simulink library "ddm"  (R2021b)
settings: Solver=VariableStepAuto  StartTime=0.0  StopTime=10.0  RelTol=1e-3
undefined symbols (not defined in the file or in its folder): ENUM_ADASACCSTA_ERROR, ENUM_ADASACCSTA_OFF, ENUM_ADASACCSTA_STANDBY, ENUM_ADASISASTA_OFF, ENUM_ALLOWMOV_ALLOWREADY, ENUM_APS, ENUM_BRKSTA_ERROR, ENUM_BRKSTA_OFF, ENUM_BRKSTA_ON, ENUM_CHGPREACTERRSTA_OBCPRE, ENUM_DCDCFAULTSTA_ANYFAULTLV1, ENUM_DCDCFAULTSTA_ANYFAULTLV2, ENUM_DRIVETRAIN_AWD, ENUM_DRIVETRAIN_FWD, ENUM_DRIVETRAIN_RWD, ENUM_DRSEATSTA_INVALID, ENUM_EDUDRTSTA_NORMAL, ENUM_EPBSTA_APPLIED, ENUM_EPBSTA_RELEASED, ENUM_HVBATTREADYPRE_READY, ENUM_MCUWARN_LV0, ENUM_MCUWARN_LV1, ENUM_MCUWARN_LV2, ENUM_MCUWARN_LV3, ENUM_MCUWARN_NOERROR, ENUM_OBCFAULTSTA_ANYFAULT, ENUM_PAS_R2F2, ENUM_PDFAULT_BATTPDFAIL, ENUM_PDFAULT_DCDCDISABLE, ENUM_PDFAULT_MCUDISABLE, ENUM_PDFAULT_MCUDISCHRG, ENUM_POWERSTA_OFF, ENUM_POWERSTA_ON, ENUM_POWERSTA_READY, ENUM_POWERSTA_STANDBY, ENUM_PRESSINDI_LOW, ENUM_PUFAULT_BATTUPFAIL, ENUM_PUFAULT_DCDCENABLEFAIL, ENUM_PUFAULT_PRECHRGCHKFAIL, ENUM_PUFAULT_SAFETYCHKFAIL, ENUM_PUSTATE_COMPLETED, ENUM_PWRSTASW_OFF, ENUM_PWRSTASW_OFFA, ENUM_PWRSTASW_OFFCHVCHRG, ENUM_PWRSTASW_OFFCLVCHRG, ENUM_PWRSTASW_ON, ENUM_PWRSTASW_ONHVCHRG, ENUM_PWRSTASW_READY, ENUM_PWRSTASW_STANDBY, ENUM_RANGESTA_12IN, ENUM_RANGESTA_12OUT, ENUM_SHIFTCOMMAND_D, ENUM_SHIFTCOMMAND_N, ENUM_SHIFTCOMMAND_P, ENUM_SHIFTCOMMAND_R, ENUM_ZONEMALFUNLV_1ST, ENUM_ZONEMALFUNLV_2ND, ENUM_ZONEMALFUNLV_3RD, ENUM_ZONEMALFUNLV_4TH, ENUM_ZONESPDCTRLMODE_ACC ... (+832)
libraries: hcu_lib x738, $bdroot x26, simulink x7
(part 4 of 25)

== system ddm/DDM/DDM/TQD ==
  VPMM_SysPwrSta_enum : Inport
  VINP_AccelPedal1Vol_V : Inport  Port=2
  VINP_AccelPedal2Vol_V : Inport  Port=3
  VDHP_EAPS12RangeSta_enum : Inport  Port=4
  VDHP_EAPCRBAD_flg : Inport  Port=5
  task_time_s : Inport  Port=6
  DTC_clear_request : Inport  Port=7
  No_CAN3_BUS_OFF : Inport  Port=8
  No_CAN1_BUS_OFF : Inport  Port=9
  VINP_CANMsgValidMCUF1_flg : Inport  Port=10
  VINP_CANMsgValidMCUR1_flg : Inport  Port=11
  VINP_CANMsgValidShifter1_flg : Inport  Port=12
  VINP_CANMsgValidESC7_flg : Inport  Port=13
  VINP_CANMsgValidESC1_flg : Inport  Port=14
  VINP_CANMsgValidESC5_flg : Inport  Port=15
  VDDM_MCUF1RCErr_flg : Inport  Port=16
  VDDM_MCUF1CSErr_flg : Inport  Port=17
  VDDM_MCUR1RCErr_flg : Inport  Port=18
  VDDM_MCUR1CSErr_flg : Inport  Port=19
  VDDM_Shifter1RCErr_flg : Inport  Port=20
  VDDM_Shifter1CSErr_flg : Inport  Port=21
  VDDM_ESC7RCErr_flg : Inport  Port=22
  VDDM_ESC7CSErr_flg : Inport  Port=23
  VDDM_ESC1RCErr_flg : Inport  Port=24
  VDDM_ESC1CSErr_flg : Inport  Port=25
  VDDM_ESC5RCErr_flg : Inport  Port=26
  VDDM_ESC5CSErr_flg : Inport  Port=27
  VINP_FrEDUDrtSta_flg : Inport  Port=28
  VINP_VehSpeed_kph : Inport  Port=29
  VINP_FrEDURealTMTq_Nm : Inport  Port=30
  VTQR_FrTMTqReq_Nm : Inport  Port=31
  VINP_RrEDUDrtSta_flg : Inport  Port=32
  VINP_RrEDURealTMTq_Nm : Inport  Port=33
  VTQR_RrTMTqReq_Nm : Inport  Port=34
  VINP_MCUWarnF_enum : Inport  Port=35
  VINP_MCUWarnR_enum : Inport  Port=36
  APS_DDM : Subsystem
  EPB : Subsystem  Commented=on
  ESC1_DDM : Subsystem
  ESC5_DDM : Subsystem
  ESC7_DDM : Subsystem
  Logical Operator{,1..5} (6 alike) : Logic  Operator=NOT  AllPortsSameDT=off  OutDataTypeStr=boolean
  MCU1_DDM : Subsystem
  MCU_DDM : Subsystem
  Shifter1_DDM : Subsystem
  VDDM_APS1SigOoRDTC_raw32 : Outport
  VDDM_APS2SigOoRDTC_raw32 : Outport  Port=2
  VDDM_APSCorrErrDTC_raw32 : Outport  Port=3
  VDDM_MCUF1NoComDTC_raw32 : Outport  Port=4
  VDDM_MCUR1NoComDTC_raw32 : Outport  Port=5
  VDDM_Shifter1NoComDTC_raw32 : Outport  Port=6
  VDDM_ESC7NoComDTC_raw32 : Outport  Port=7
  VDDM_ESC1NoComDTC_raw32 : Outport  Port=8
  VDDM_ESC5NoComDTC_raw32 : Outport  Port=9
  VDDM_MCUF1RCErrDTC_raw32 : Outport  Port=10
  VDDM_MCUR1RCErrDTC_raw32 : Outport  Port=11
  VDDM_MCUF1CSErrDTC_raw32 : Outport  Port=12
  VDDM_MCUR1CSErrDTC_raw32 : Outport  Port=13
  VDDM_Shifter1RCErrDTC_raw32 : Outport  Port=14
  VDDM_Shifter1CSErrDTC_raw32 : Outport  Port=15
  VDDM_ESC7RCErrDTC_raw32 : Outport  Port=16
  VDDM_ESC7CSErrDTC_raw32 : Outport  Port=17
  VDDM_ESC1RCErrDTC_raw32 : Outport  Port=18
  VDDM_ESC1CSErrDTC_raw32 : Outport  Port=19
  VDDM_ESC5RCErrDTC_raw32 : Outport  Port=20
  VDDM_ESC5CSErrDTC_raw32 : Outport  Port=21
  VDDM_FrMCUTqErrDTC_raw32 : Outport  Port=22
  VDDM_RrMCUTqErrDTC_raw32 : Outport  Port=23
  VDDM_MCUF1NoComCFS_flg : Outport  Port=24
  VDDM_MCUF1RCErrCFS_flg : Outport  Port=25
  VDDM_MCUF1CSErrCFS_flg : Outport  Port=26
  VDDM_MCUR1NoComCFS_flg : Outport  Port=27
  VDDM_MCUR1RCErrCFS_flg : Outport  Port=28
  VDDM_MCUR1CSErrCFS_flg : Outport  Port=29
  VDDM_ESC7NoComCFS_flg : Outport  Port=30
  VDDM_ESC7RCErrCFS_flg : Outport  Port=31
  VDDM_ESC7CSErrCFS_flg : Outport  Port=32
  VDDM_ESC1NoComCFS_flg : Outport  Port=33
  VDDM_ESC1RCErrCFS_flg : Outport  Port=34
  VDDM_ESC1CSErrCFS_flg : Outport  Port=35
  VDDM_ESC5NoComCFS_flg : Outport  Port=36
  VDDM_ESC5RCErrCFS_flg : Outport  Port=37
  VDDM_ESC5CSErrCFS_flg : Outport  Port=38
  wires:
  VINP_AccelPedal2Vol_V/1 -> [VINP_AccelPedal2Vol_V]
  VDHP_EAPS12RangeSta_enum/1 -> [VDHP_EAPS12RangeSta_enum]
  VDHP_EAPCRBAD_flg/1 -> [VDHP_EAPCRBAD_flg]
  VINP_AccelPedal1Vol_V/1 -> [VINP_AccelPedal1Vol_V]
  VPMM_SysPwrSta_enum/1 -> [VPMM_SysPwrSta_enum]
  [VDHP_EAPCRBAD_flg] -> APS_DDM/5(VDHP_EAPCRBAD_flg)
  [VPMM_SysPwrSta_enum] -> APS_DDM/1(VPMM_SysPwrSta_enum)
  [VINP_AccelPedal1Vol_V] -> APS_DDM/2(VINP_AccelPedal1Vol_V)
  [VINP_AccelPedal2Vol_V] -> APS_DDM/3(VINP_AccelPedal2Vol_V)
  [VDHP_EAPS12RangeSta_enum] -> APS_DDM/4(VDHP_EAPS12RangeSta_enum)
  APS_DDM/1(VDDM_APS1SigOoRDTC_raw32) -> VDDM_APS1SigOoRDTC_raw32/1
  APS_DDM/2(VDDM_APS2SigOoRDTC_raw32) -> VDDM_APS2SigOoRDTC_raw32/1
  APS_DDM/3(VDDM_APSCorrErrDTC_raw32) -> VDDM_APSCorrErrDTC_raw32/1
  task_time_s/1 -> [task_time_s]
  [task_time_s] -> APS_DDM/6(task_time_s)
  DTC_clear_request/1 -> [DTC_clear_request]
  [DTC_clear_request] -> APS_DDM/7(DTC_clear_request)
  [task_time_s] -> MCU1_DDM/1(task_time_s)
  [task_time_s] -> Shifter1_DDM/1(task_time_s)
  [task_time_s] -> ESC7_DDM/1(task_time_s)
  [VPMM_SysPwrSta_enum] -> MCU1_DDM/2(VPMM_SysPwrSta_enum)
  [No_CAN3_BUS_OFF] -> MCU1_DDM/3(No_CAN3_BUS_OFF)
  [VDDM_MCUF1NoCom_flg] -> MCU1_DDM/4(VDDM_MCUF1NoCom_flg)
  [VDDM_MCUR1NoCom_flg] -> MCU1_DDM/5(VDDM_MCUR1NoCom_flg)
  [DTC_clear_request] -> MCU1_DDM/10(DTC_clear_request)
  [VPMM_SysPwrSta_enum] -> Shifter1_DDM/2(VPMM_SysPwrSta_enum)
  [No_CAN3_BUS_OFF] -> Shifter1_DDM/3(No_CAN3_BUS_OFF)
  [VDDM_Shifter1NoCom_flg] -> Shifter1_DDM/4(VDDM_Shifter1NoCom_flg)
  [DTC_clear_request] -> Shifter1_DDM/7(DTC_clear_request)
  [VDDM_ESC7NoCom_flg] -> ESC7_DDM/4(VDDM_ESC7NoCom_flg)
  [No_CAN1_BUS_OFF] -> ESC7_DDM/3(No_CAN1_BUS_OFF)
  [VPMM_SysPwrSta_enum] -> ESC7_DDM/2(VPMM_SysPwrSta_enum)
  [DTC_clear_request] -> ESC7_DDM/7(DTC_clear_request)
  [task_time_s] -> ESC1_DDM/1(task_time_s)
  [VPMM_SysPwrSta_enum] -> ESC1_DDM/2(VPMM_SysPwrSta_enum)
  [No_CAN1_BUS_OFF] -> ESC1_DDM/3(No_CAN1_BUS_OFF)
  [VDDM_ESC1NoCom_flg] -> ESC1_DDM/4(VDDM_ESC1NoCom_flg)
  [DTC_clear_request] -> ESC1_DDM/7(DTC_clear_request)
  [task_time_s] -> ESC5_DDM/1(task_time_s)
  [VPMM_SysPwrSta_enum] -> ESC5_DDM/2(VPMM_SysPwrSta_enum)
  [No_CAN1_BUS_OFF] -> ESC5_DDM/3(No_CAN1_BUS_OFF)
  [VDDM_ESC5NoCom_flg] -> ESC5_DDM/4(VDDM_ESC5NoCom_flg)
  [DTC_clear_request] -> ESC5_DDM/7(DTC_clear_request)
  MCU1_DDM/1(VDDM_MCUF1NoComDTC_raw32) -> VDDM_MCUF1NoComDTC_raw32/1
  MCU1_DDM/2(VDDM_MCUR1NoComDTC_raw32) -> VDDM_MCUR1NoComDTC_raw32/1
  Shifter1_DDM/1(VDDM_Shifter1NoComDTC_raw32) -> VDDM_Shifter1NoComDTC_raw32/1
  ESC1_DDM/1(VDDM_ESC1NoComDTC_raw32) -> VDDM_ESC1NoComDTC_raw32/1
  ESC5_DDM/1(VDDM_ESC5NoComDTC_raw32) -> VDDM_ESC5NoComDTC_raw32/1
  No_CAN3_BUS_OFF/1 -> [No_CAN3_BUS_OFF]
  No_CAN1_BUS_OFF/1 -> [No_CAN1_BUS_OFF]
  VINP_CANMsgValidMCUF1_flg/1 -> Logical Operator5/1
  VINP_CANMsgValidMCUR1_flg/1 -> Logical Operator4/1
  VINP_CANMsgValidShifter1_flg/1 -> Logical Operator3/1
  VINP_CANMsgValidESC7_flg/1 -> Logical Operator2/1
  VINP_CANMsgValidESC1_flg/1 -> Logical Operator1/1
  VINP_CANMsgValidESC5_flg/1 -> Logical Operator/1
  Logical Operator/1 -> [VDDM_ESC5NoCom_flg]
  Logical Operator1/1 -> [VDDM_ESC1NoCom_flg]
  Logical Operator2/1 -> [VDDM_ESC7NoCom_flg]
  Logical Operator3/1 -> [VDDM_Shifter1NoCom_flg]
  Logical Operator4/1 -> [VDDM_MCUR1NoCom_flg]
  Logical Operator5/1 -> [VDDM_MCUF1NoCom_flg]
  [VDDM_MCUF1RCErr_flg] -> MCU1_DDM/6(VDDM_MCUF1RCErr_flg)
  [VDDM_MCUF1CSErr_flg] -> MCU1_DDM/7(VDDM_MCUF1CSErr_flg)
  [VDDM_MCUR1RCErr_flg] -> MCU1_DDM/8(VDDM_MCUR1RCErr_flg)
  [VDDM_MCUR1CSErr_flg] -> MCU1_DDM/9(VDDM_MCUR1CSErr_flg)
  ESC7_DDM/1(VDDM_ESC7NoComDTC_raw32) -> VDDM_ESC7NoComDTC_raw32/1
  MCU1_DDM/4(VDDM_MCUR1RCErrDTC_raw32) -> VDDM_MCUR1RCErrDTC_raw32/1
  MCU1_DDM/3(VDDM_MCUF1RCErrDTC_raw32) -> VDDM_MCUF1RCErrDTC_raw32/1
  MCU1_DDM/5(VDDM_MCUF1CSErrDTC_raw32) -> VDDM_MCUF1CSErrDTC_raw32/1
  MCU1_DDM/6(VDDM_MCUR1CSErrDTC_raw32) -> VDDM_MCUR1CSErrDTC_raw32/1
  Shifter1_DDM/2(VDDM_Shifter1RCErrDTC_raw32) -> VDDM_Shifter1RCErrDTC_raw32/1
  Shifter1_DDM/3(VDDM_Shifter1CSErrDTC_raw32) -> VDDM_Shifter1CSErrDTC_raw32/1
  ESC7_DDM/2(VDDM_ESC7RCErrDTC_raw32) -> VDDM_ESC7RCErrDTC_raw32/1
  ESC7_DDM/3(VDDM_ESC7CSErrDTC_raw32) -> VDDM_ESC7CSErrDTC_raw32/1
  ESC1_DDM/3(VDDM_ESC1CSErrDTC_raw32) -> VDDM_ESC1CSErrDTC_raw32/1
  ESC1_DDM/2(VDDM_ESC1RCErrDTC_raw32) -> VDDM_ESC1RCErrDTC_raw32/1
  ESC5_DDM/2(VDDM_ESC5RCErrDTC_raw32) -> VDDM_ESC5RCErrDTC_raw32/1
  ESC5_DDM/3(VDDM_ESC5CSErrDTC_raw32) -> VDDM_ESC5CSErrDTC_raw32/1
  MCU_DDM/2(VDDM_RrMCUTqErrDTC_raw32) -> VDDM_RrMCUTqErrDTC_raw32/1
  MCU_DDM/1(VDDM_FrMCUTqErrDTC_raw32) -> VDDM_FrMCUTqErrDTC_raw32/1
  [VDDM_Shifter1RCErr_flg] -> Shifter1_DDM/5(VDDM_Shifter1RCErr_flg)
  [VDDM_Shifter1CSErr_flg] -> Shifter1_DDM/6(VDDM_Shifter1CSErr_flg)
  VDDM_MCUR1RCErr_flg/1 -> [VDDM_MCUR1RCErr_flg]
  VDDM_MCUR1CSErr_flg/1 -> [VDDM_MCUR1CSErr_flg]
  VDDM_MCUF1CSErr_flg/1 -> [VDDM_MCUF1CSErr_flg]
  VDDM_MCUF1RCErr_flg/1 -> [VDDM_MCUF1RCErr_flg]
  VDDM_Shifter1RCErr_flg/1 -> [VDDM_Shifter1RCErr_flg]
  VDDM_Shifter1CSErr_flg/1 -> [VDDM_Shifter1CSErr_flg]
  [VDDM_ESC7RCErr_flg] -> ESC7_DDM/5(VDDM_ESC7RCErr_flg)
  [VDDM_ESC7CSErr_flg] -> ESC7_DDM/6(VDDM_ESC7CSErr_flg)
  VDDM_ESC7CSErr_flg/1 -> [VDDM_ESC7CSErr_flg]
  VDDM_ESC7RCErr_flg/1 -> [VDDM_ESC7RCErr_flg]
  [VDDM_ESC1RCErr_flg] -> ESC1_DDM/5(VDDM_ESC1RCErr_flg)
  [VDDM_ESC1CSErr_flg] -> ESC1_DDM/6(VDDM_ESC1CSErr_flg)
  VDDM_ESC1CSErr_flg/1 -> [VDDM_ESC1CSErr_flg]
  VDDM_ESC1RCErr_flg/1 -> [VDDM_ESC1RCErr_flg]
  [VDDM_ESC5RCErr_flg] -> ESC5_DDM/5(VDDM_ESC5RCErr_flg)
  [VDDM_ESC5CSErr_flg] -> ESC5_DDM/6(VDDM_ESC5CSErr_flg)
  VDDM_ESC5CSErr_flg/1 -> [VDDM_ESC5CSErr_flg]
  VDDM_ESC5RCErr_flg/1 -> [VDDM_ESC5RCErr_flg]
  VINP_RrEDURealTMTq_Nm/1 -> [VINP_RrEDURealTMTq_Nm]
  VINP_FrEDUDrtSta_flg/1 -> [VINP_FrEDUDrtSta_flg]
  VTQR_RrTMTqReq_Nm/1 -> [VTQR_RrTMTqReq_Nm]
  VINP_FrEDURealTMTq_Nm/1 -> [VINP_FrEDURealTMTq_Nm]
  VTQR_FrTMTqReq_Nm/1 -> [VTQR_FrTMTqReq_Nm]
  VINP_RrEDUDrtSta_flg/1 -> [VINP_RrEDUDrtSta_flg]
  VINP_VehSpeed_kph/1 -> [VINP_VehSpeed_kph]
  ESC7_DDM/6(VDDM_ESC7CSErrCFS_flg) -> VDDM_ESC7CSErrCFS_flg/1
  ESC7_DDM/5(VDDM_ESC7RCErrCFS_flg) -> VDDM_ESC7RCErrCFS_flg/1
  ESC7_DDM/4(VDDM_ESC7NoComCFS_flg) -> VDDM_ESC7NoComCFS_flg/1
  ESC5_DDM/6(VDDM_ESC5CSErrCFS_flg) -> VDDM_ESC5CSErrCFS_flg/1
  ESC5_DDM/4(VDDM_ESC5NoComCFS_flg) -> VDDM_ESC5NoComCFS_flg/1
  ESC1_DDM/5(VDDM_ESC1RCErrCFS_flg) -> VDDM_ESC1RCErrCFS_flg/1
  ESC5_DDM/5(VDDM_ESC5RCErrCFS_flg) -> VDDM_ESC5RCErrCFS_flg/1
  ESC1_DDM/4(VDDM_ESC1NoComCFS_flg) -> VDDM_ESC1NoComCFS_flg/1
  ESC1_DDM/6(VDDM_ESC1CSErrCFS_flg) -> VDDM_ESC1CSErrCFS_flg/1
  VINP_MCUWarnF_enum/1 -> [VINP_MCUWarnF_enum]
  VINP_MCUWarnR_enum/1 -> [VINP_MCUWarnR_enum]
  MCU1_DDM/12(VDDM_MCUR1CSErrCFS_flg) -> [VDDM_MCUR1CSErrCFS_flg]
  MCU1_DDM/8(VDDM_MCUF1RCErrCFS_flg) -> [VDDM_MCUF1RCErrCFS_flg]
  MCU1_DDM/9(VDDM_MCUF1CSErrCFS_flg) -> [VDDM_MCUF1CSErrCFS_flg]
  MCU1_DDM/10(VDDM_MCUR1NoComCFS_flg) -> [VDDM_MCUR1NoComCFS_flg]
  MCU1_DDM/7(VDDM_MCUF1NoComCFS_flg) -> [VDDM_MCUF1NoComCFS_flg]
  MCU1_DDM/11(VDDM_MCUR1RCErrCFS_flg) -> [VDDM_MCUR1RCErrCFS_flg]
  [VDDM_MCUF1NoComCFS_flg] -> VDDM_MCUF1NoComCFS_flg/1
  [VDDM_MCUR1CSErrCFS_flg] -> VDDM_MCUR1CSErrCFS_flg/1
  [VDDM_MCUF1CSErrCFS_flg] -> VDDM_MCUF1CSErrCFS_flg/1
  [VDDM_MCUR1NoComCFS_flg] -> VDDM_MCUR1NoComCFS_flg/1
  [VDDM_MCUR1RCErrCFS_flg] -> VDDM_MCUR1RCErrCFS_flg/1
  [VDDM_MCUF1RCErrCFS_flg] -> VDDM_MCUF1RCErrCFS_flg/1
  [VINP_VehSpeed_kph] -> MCU_DDM/7(VINP_VehSpeed_kph)
  [VINP_MCUWarnR_enum] -> MCU_DDM/18(VINP_MCUWarnR_enum)
  [VDDM_MCUR1NoComCFS_flg] -> MCU_DDM/11(VDDM_MCUR1NoComCFS_flg)
  [DTC_clear_request] -> MCU_DDM/19(DTC_clear_request)
  [VINP_RrEDURealTMTq_Nm] -> MCU_DDM/15(VINP_RrEDURealTMTq_Nm)
  [VINP_FrEDURealTMTq_Nm] -> MCU_DDM/9(VINP_FrEDURealTMTq_Nm)
  [VINP_FrEDUDrtSta_flg] -> MCU_DDM/8(VINP_FrEDUDrtSta_flg)
  [VTQR_RrTMTqReq_Nm] -> MCU_DDM/16(VTQR_RrTMTqReq_Nm)
  [task_time_s] -> MCU_DDM/1(task_time_s)
  [VTQR_FrTMTqReq_Nm] -> MCU_DDM/10(VTQR_FrTMTqReq_Nm)
  [VDDM_MCUF1NoComCFS_flg] -> MCU_DDM/4(VDDM_MCUF1NoComCFS_flg)
  [VPMM_SysPwrSta_enum] -> MCU_DDM/2(VPMM_SysPwrSta_enum)
  [VDDM_MCUR1CSErrCFS_flg] -> MCU_DDM/13(VDDM_MCUR1CSErrCFS_flg)
  [VINP_RrEDUDrtSta_flg] -> MCU_DDM/14(VINP_RrEDUDrtSta_flg)
  [VINP_MCUWarnF_enum] -> MCU_DDM/17(VINP_MCUWarnF_enum)
  [No_CAN3_BUS_OFF] -> MCU_DDM/3(No_CAN3_BUS_OFF)
  [VDDM_MCUF1CSErrCFS_flg] -> MCU_DDM/6(VDDM_MCUF1CSErrCFS_flg)
  [VDDM_MCUF1RCErrCFS_flg] -> MCU_DDM/5(VDDM_MCUF1RCErrCFS_flg)
  [VDDM_MCUR1RCErrCFS_flg] -> MCU_DDM/12(VDDM_MCUR1RCErrCFS_flg)

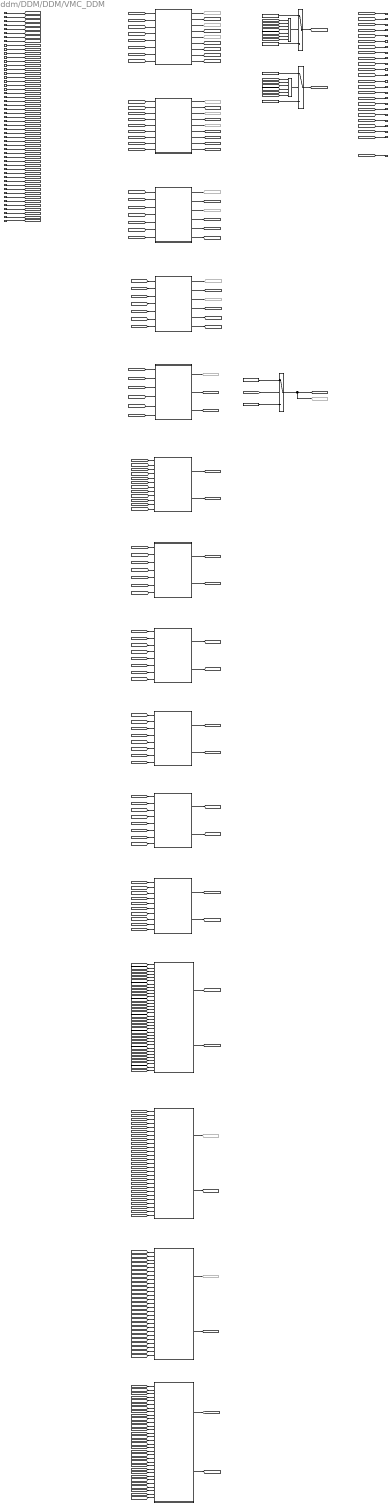
== system ddm/DDM/DDM/VMC_DDM ==
  note: FCM2
  note: BMS
  note: FCM3
  note: FCM4
  note: FCM5
  note: ZoneSCP
  note: FCMACC
  note: MCU_Fr
  note: MCU_Rr
  note: CCU
  note: ACC Accel
  note: ACC Malfunction
  note: CC Malfunction
  note: MSA Malfunction
  note: ISA Malfunction
  task_time_s : Inport
  VDDM_FCM2NoCom_flg : Inport  Port=2
  VDDM_FCM2RCErr_flg : Inport  Port=3
  VDDM_FCM2CSErr_flg : Inport  Port=4
  No_CAN_BUS_OFF : Inport  Port=5
  VPMM_PowerSta_enum : Inport  Port=6
  VINP_ADASACCSta_enum : Inport  Port=7
  DTC_clear_request : Inport  Port=8
  VDDM_FCM3NoCom_flg : Inport  Port=9
  VDDM_FCM3RCErr_flg : Inport  Port=10
  VDDM_FCM3CSErr_flg : Inport  Port=11
  VINP_ADASISASta_enum : Inport  Port=12
  VDDM_FCM4NoCom_flg : Inport  Port=13
  VDDM_FCM4CSErr_flg : Inport  Port=14
  VDDM_FCM5NoCom_flg : Inport  Port=15
  VDDM_FCM5CSErr_flg : Inport  Port=16
  VDDM_C3BMS6LCCFS_flg : Inport  Port=17
  VDDM_C3BMS6RCCFS_flg : Inport  Port=18
  VDDM_C3BMS6CSCFS_flg : Inport  Port=19
  VINP_BMSWarn8_flg : Inport  Port=20
  VINP_BMSWarn7_flg : Inport  Port=21
  VINP_BMSWarn6_flg : Inport  Port=22
  VINP_BMSWarn5_flg : Inport  Port=23
  VINP_BMSWarn4_flg : Inport  Port=24
  VDDM_ZoneSCPNoCom_flg : Inport  Port=25
  VINP_VehSpeed_kph : Inport  Port=26
  VDDM_MCUF1NoComCFS_flg : Inport  Port=27
  VDDM_MCUF1RCErrCFS_flg : Inport  Port=28
  VDDM_MCUF1CSErrCFS_flg : Inport  Port=29
  VINP_MCUWarnF_enum : Inport  Port=30
  VINP_MCUWarnR_enum : Inport  Port=31
  VDDM_MCUR1NoComCFS_flg : Inport  Port=32
  VDDM_MCUR1RCErrCFS_flg : Inport  Port=33
  VDDM_MCUR1CSErrCFS_flg : Inport  Port=34
  VDDM_C3CCU2LCCFS_flg : Inport  Port=35
  VDDM_C3CCU2RCCFS_flg : Inport  Port=36
  VDDM_C3CCU2CSCFS_flg : Inport  Port=37
  VINP_DCDCFaultSta_enum : Inport  Port=38
  VVMC_ADASActive_flg : Inport  Port=39
  VINP_ACCRequireAccel_mps2 : Inport  Port=40
  VDDM_ESC7NoComCFS_flg : Inport  Port=41
  VDDM_ESC7RCErrCFS_flg : Inport  Port=42
  VDDM_ESC7CSErrCFS_flg : Inport  Port=43
  VDDM_ESC1NoComCFS_flg : Inport  Port=44
  VDDM_ESC1RCErrCFS_flg : Inport  Port=45
  VDDM_ESC1CSErrCFS_flg : Inport  Port=46
  VDDM_ESC5NoComCFS_flg : Inport  Port=47
  VDDM_ESC5RCErrCFS_flg : Inport  Port=48
  VDDM_ESC5CSErrCFS_flg : Inport  Port=49
  VINP_ZoneSpdCtrlMode_enum : Inport  Port=50
  No_CAN1_BUS_OFF : Inport  Port=51
  No_CAN3_BUS_OFF : Inport  Port=52
  No_CAN4_BUS_OFF : Inport  Port=53
  ACC Acceleration Command Error : Subsystem
  "ACC Malfunction " : Subsystem
  "BMS Signal Error " : Subsystem
  "CC Malfunction " : Subsystem
  CCU Signal Error : Subsystem
  Constant1 : Constant  Value=TRUE
  Constant2 : Constant  Value=TRUE
  Constant21 : Constant  Value=FALSE
  Constant3 : Constant  Value=FALSE
  Constant4 : Constant  Value=TRUE
  Constant5 : Constant  Value=FALSE
  FCM2 : Subsystem
  FCM3 : Subsystem
  FCM4 : Subsystem
  FCM5 : Subsystem
  FCMACC Signal Error : Subsystem
  Goto12 : Goto  Commented=on  GotoTag=VDDM_FCM2NoComDFS_flg
  Goto13 : Goto  Commented=on  GotoTag=VDDM_FCM2RCErrDFS_flg
  Goto14 : Goto  Commented=on  GotoTag=VDDM_FCM2CSErrDFS_flg
  Goto15 : Goto  Commented=on  GotoTag=VDDM_FCM3NoComDFS_flg
  Goto16 : Goto  Commented=on  GotoTag=VDDM_FCM3RCErrDFS_flg
  Goto17 : Goto  Commented=on  GotoTag=VDDM_FCM3CSErrDFS_flg
  Goto18 : Goto  Commented=on  GotoTag=VDDM_FCM4NoComDFS_flg
  Goto19 : Goto  Commented=on  GotoTag=VDDM_FCM4CSErrDFS_flg
  Goto20 : Goto  Commented=on  GotoTag=VDDM_FCM5NoComDFS_flg
  Goto21 : Goto  Commented=on  GotoTag=VDDM_FCM5CSErrDFS_flg
  Goto48 : Goto  Commented=on  GotoTag=VDDM_ZoneSCPNoComDFS_flg
  Goto50 : Goto  Commented=on  GotoTag=VDDM_ZoneDRSCPComErr_flg
  Goto86 : Goto  Commented=on  GotoTag=VDDM_CCMalfuncCFS_flg
  Goto87 : Goto  Commented=on  GotoTag=VDDM_MSAMalfuncCFS_flg
  "ISA Malfunction " : Subsystem
  Logical Operator1 : Logic  Operator=OR  Inputs=6  AllPortsSameDT=off  OutDataTypeStr=boolean
  Logical Operator2 : Logic  Operator=OR  Inputs=7  AllPortsSameDT=off  OutDataTypeStr=boolean
  MCU_Fr Signal Error : Subsystem
  MCU_Rr Signal Error : Subsystem
  "MSA Malfunction " : Subsystem
  Switch : Switch  Criteria=u2 ~= 0
  Switch1 : Switch  Criteria=u2 ~= 0
  Switch2 : Switch  Criteria=u2 ~= 0
  ZoneSCP : Subsystem
  VDDM_FCM2NoComDTC_raw32 : Outport
  VDDM_FCM2RCErrDTC_raw32 : Outport  Port=2
  VDDM_FCM2CSErrDTC_raw32 : Outport  Port=3
  VDDM_FCM3NoComDTC_raw32 : Outport  Port=4
  VDDM_FCM3RCErrDTC_raw32 : Outport  Port=5
  VDDM_FCM3CSErrDTC_raw32 : Outport  Port=6
  VDDM_FCM4NoComDTC_raw32 : Outport  Port=7
  VDDM_FCM4CSErrDTC_raw32 : Outport  Port=8
  VDDM_FCM5NoComDTC_raw32 : Outport  Port=9
  VDDM_FCM5CSErrDTC_raw32 : Outport  Port=10
  VDDM_ZoneSCPNoComDTC_raw32 : Outport  Port=11
  VDDM_BMSSigErrDetDTC_raw32 : Outport  Port=12
  VDDM_FCMACCSigErrDetDTC_raw32 : Outport  Port=13
  VDDM_FrMCUSigErrDetDTC_raw32 : Outport  Port=14
  VDDM_RrMCUSigErrDetDTC_raw32 : Outport  Port=15
  VDDM_CCUSigErrDetDTC_raw32 : Outport  Port=16
  VDDM_ACCAccelCmdErrDetDTC_raw32 : Outport  Port=17
  VDDM_ACCMalfuncDetDTC_raw32 : Outport  Port=18
  VDDM_CCMalfuncDetDTC_raw32 : Outport  Port=19
  VDDM_MSAMalfuncDetDTC_raw32 : Outport  Port=20
  VDDM_ISAMalfuncDetDTC_raw32 : Outport  Port=21
  VDDM_VCUACCErr_flg : Outport  Port=22
  VDDM_VCUISAErr_flg : Outport  Port=23
  VDDM_EDriveSysErrVMC_flg : Outport  Port=24
  wires:
  VDDM_FCM5CSErr_flg/1 -> [VDDM_FCM5CSErr_flg]
  VDDM_FCM5NoCom_flg/1 -> [VDDM_FCM5NoCom_flg]
  VDDM_FCM4CSErr_flg/1 -> [VDDM_FCM4CSErr_flg]
  VDDM_FCM3CSErr_flg/1 -> [VDDM_FCM3CSErr_flg]
  VDDM_C3BMS6CSCFS_flg/1 -> [VDDM_C3BMS6CSCFS_flg]
  VINP_ADASISASta_enum/1 -> [VINP_ADASISASta_enum]
  VDDM_FCM2RCErr_flg/1 -> [VDDM_FCM2RCErr_flg]
  VPMM_PowerSta_enum/1 -> [VPMM_PowerSta_enum]
  No_CAN_BUS_OFF/1 -> [No_CAN_BUS_OFF]
  [VPMM_PowerSta_enum] -> FCM5/5(VPMM_PowerSta_enum)
  [No_CAN_BUS_OFF] -> FCM5/4(No_CAN_BUS_OFF)
  [DTC_clear_request] -> FCM5/7(DTC_clear_request)
  [VINP_ADASISASta_enum] -> FCM5/6(VINP_ADASISASta_enum)
  [task_time_s] -> FCM5/1(task_time_s)
  [VDDM_FCM5NoCom_flg] -> FCM5/2(VDDM_FCM5NoCom_flg)
  [VDDM_FCM5CSErr_flg] -> FCM5/3(VDDM_FCM5CSErr_flg)
  VINP_BMSWarn7_flg/1 -> [VINP_BMSWarn7_flg]
  [task_time_s] -> "BMS Signal Error "/1(task_time_s)
  [DTC_clear_request] -> FCM4/7(DTC_clear_request)
  [VDDM_FCM4CSErr_flg] -> FCM4/3(VDDM_FCM4CSErr_flg)
  VDDM_FCM2NoCom_flg/1 -> [VDDM_FCM2NoCom_flg]
  [VINP_BMSWarn5_flg] -> "BMS Signal Error "/10(VINP_BMSWarn5_flg)
  [VINP_BMSWarn4_flg] -> "BMS Signal Error "/11(VINP_BMSWarn4_flg)
  [DTC_clear_request] -> "BMS Signal Error "/12(DTC_clear_request)
  [VPMM_PowerSta_enum] -> "BMS Signal Error "/6(VPMM_PowerSta_enum)
  [VINP_BMSWarn7_flg] -> "BMS Signal Error "/8(VINP_BMSWarn7_flg)
  [VINP_BMSWarn8_flg] -> "BMS Signal Error "/7(VINP_BMSWarn8_flg)
  [VDDM_C3BMS6RCCFS_flg] -> "BMS Signal Error "/3(VDDM_C3BMS6RCCFS_flg)
  [No_CAN_BUS_OFF] -> "BMS Signal Error "/5(No_CAN_BUS_OFF)
  [VDDM_C3BMS6CSCFS_flg] -> "BMS Signal Error "/4(VDDM_C3BMS6CSCFS_flg)
  [VDDM_C3BMS6LCCFS_flg] -> "BMS Signal Error "/2(VDDM_C3BMS6LCCFS_flg)
  VDDM_FCM3NoCom_flg/1 -> [VDDM_FCM3NoCom_flg]
  VDDM_C3BMS6LCCFS_flg/1 -> [VDDM_C3BMS6LCCFS_flg]
  VINP_BMSWarn5_flg/1 -> [VINP_BMSWarn5_flg]
  VINP_ADASACCSta_enum/1 -> [VINP_ADASACCSta_enum]
  [task_time_s] -> FCM4/1(task_time_s)
  VINP_BMSWarn6_flg/1 -> [VINP_BMSWarn6_flg]
  VDDM_FCM2CSErr_flg/1 -> [VDDM_FCM2CSErr_flg]
  VDDM_FCM3RCErr_flg/1 -> [VDDM_FCM3RCErr_flg]
  [VPMM_PowerSta_enum] -> FCM3/6(VPMM_PowerSta_enum)
  [VDDM_FCM3NoCom_flg] -> FCM3/2(VDDM_FCM3NoCom_flg)
  [VDDM_FCM3CSErr_flg] -> FCM3/4(VDDM_FCM3CSErr_flg)
  [DTC_clear_request] -> FCM3/9(DTC_clear_request)
  "BMS Signal Error "/1(VDDM_BMSSigErrCFS_flg) -> [VDDM_BMSSigErrCFS_flg]
  Logical Operator1/1 -> Switch1/2
  [VDDM_FCM4NoCom_flg] -> FCM4/2(VDDM_FCM4NoCom_flg)
  FCM5/2(VDDM_FCM5NoComCFS_flg) -> [VDDM_FCM5NoComCFS_flg]
  [VDDM_FCM2RCErr_flg] -> FCM2/3(VDDM_FCM2RCErr_flg)
  [No_CAN_BUS_OFF] -> FCM2/5(No_CAN_BUS_OFF)
  FCM5/1(VDDM_FCM5NoComDFS_flg) -> Goto20/1
  FCM4/1(VDDM_FCM4NoComDFS_flg) -> Goto18/1
  FCM3/3(VDDM_FCM3RCErrDFS_flg) -> Goto16/1
  FCM3/5(VDDM_FCM3CSErrDFS_flg) -> Goto17/1
  FCM2/5(VDDM_FCM2CSErrDFS_flg) -> Goto14/1
  FCM4/4(VDDM_FCM4CSErrCFS_flg) -> [VDDM_FCM4CSErrCFS_flg]
  [VPMM_PowerSta_enum] -> FCM4/5(VPMM_PowerSta_enum)
  Switch1/1 -> [VDDM_VCUISAErr_flg]
  [VDDM_FCM2NoCom_flg] -> FCM2/2(VDDM_FCM2NoCom_flg)
  [VDDM_FCM5NoComCFS_flg] -> Logical Operator1/4
  [VINP_BMSWarn6_flg] -> "BMS Signal Error "/9(VINP_BMSWarn6_flg)
  FCM3/1(VDDM_FCM3NoComDFS_flg) -> Goto15/1
  FCM2/4(VDDM_FCM2RCErrCFS_flg) -> [VDDM_FCM2RCErrCFS_flg]
  [VINP_ADASACCSta_enum] -> FCM2/7(VINP_ADASACCSta_enum)
  FCM4/3(VDDM_FCM4CSErrDFS_flg) -> Goto19/1
  Constant3/1 -> Switch1/3
  VINP_BMSWarn8_flg/1 -> [VINP_BMSWarn8_flg]
  [VDDM_FCM5CSErrCFS_flg] -> Logical Operator1/5
  [VDDM_FCM2NoComCFS_flg] -> Logical Operator2/1
  FCM5/4(VDDM_FCM5CSErrCFS_flg) -> [VDDM_FCM5CSErrCFS_flg]
  [VDDM_FCM2CSErr_flg] -> FCM2/4(VDDM_FCM2CSErr_flg)
  FCM2/2(VDDM_FCM2NoComCFS_flg) -> [VDDM_FCM2NoComCFS_flg]
  [VDDM_FCM4CSErrCFS_flg] -> Logical Operator2/5
  [VDDM_FCM3NoComCFS_flg] -> Logical Operator1/1
  [VDDM_FCM3RCErrCFS_flg] -> Logical Operator1/2
  [VDDM_FCM3CSErrCFS_flg] -> Logical Operator1/3
  [task_time_s] -> FCM2/1(task_time_s)
  [VPMM_PowerSta_enum] -> FCM2/6(VPMM_PowerSta_enum)
  FCM2/6(VDDM_FCM2CSErrCFS_flg) -> [VDDM_FCM2CSErrCFS_flg]
  [DTC_clear_request] -> FCM2/8(DTC_clear_request)
  FCM3/6(VDDM_FCM3CSErrCFS_flg) -> [VDDM_FCM3CSErrCFS_flg]
  [No_CAN_BUS_OFF] -> FCM4/4(No_CAN_BUS_OFF)
  FCM3/4(VDDM_FCM3RCErrCFS_flg) -> [VDDM_FCM3RCErrCFS_flg]
  [VINP_ADASACCSta_enum] -> FCM4/6(VINP_ADASACCSta_enum)
  FCM4/2(VDDM_FCM4NoComCFS_flg) -> [VDDM_FCM4NoComCFS_flg]
  FCM3/2(VDDM_FCM3NoComCFS_flg) -> [VDDM_FCM3NoComCFS_flg]
  Constant2/1 -> Switch1/1
  FCM2/3(VDDM_FCM2RCErrDFS_flg) -> Goto13/1
  [VDDM_FCM2CSErrCFS_flg] -> Logical Operator2/3
  Constant21/1 -> Switch/3
  Logical Operator2/1 -> Switch/2
  FCM2/1(VDDM_FCM2NoComDFS_flg) -> Goto12/1
  [VDDM_FCM2RCErrCFS_flg] -> Logical Operator2/2
  [task_time_s] -> FCM3/1(task_time_s)
  DTC_clear_request/1 -> [DTC_clear_request]
  VINP_BMSWarn4_flg/1 -> [VINP_BMSWarn4_flg]
  [VINP_ADASISASta_enum] -> FCM3/8(VINP_ADASISASta_enum)
  [VDDM_FCM4NoComCFS_flg] -> Logical Operator2/4
  VDDM_C3BMS6RCCFS_flg/1 -> [VDDM_C3BMS6RCCFS_flg]
  VDDM_FCM4NoCom_flg/1 -> [VDDM_FCM4NoCom_flg]
  [VINP_ADASACCSta_enum] -> FCM3/7(VINP_ADASACCSta_enum)
  Switch/1 -> [VDDM_VCUACCErr_flg]
  Constant1/1 -> Switch/1
  FCM5/3(VDDM_FCM5CSErrDFS_flg) -> Goto21/1
  task_time_s/1 -> [task_time_s]
  [VDDM_FCM3RCErr_flg] -> FCM3/3(VDDM_FCM3RCErr_flg)
  [No_CAN_BUS_OFF] -> FCM3/5(No_CAN_BUS_OFF)
  [VDDM_FCM2CSErrDTC_raw32] -> VDDM_FCM2CSErrDTC_raw32/1
  [VDDM_FCM3NoComDTC_raw32] -> VDDM_FCM3NoComDTC_raw32/1
  [VDDM_FCM2NoComDTC_raw32] -> VDDM_FCM2NoComDTC_raw32/1
  [VDDM_FCM3CSErrDTC_raw32] -> VDDM_FCM3CSErrDTC_raw32/1
  [VDDM_FCM2RCErrDTC_raw32] -> VDDM_FCM2RCErrDTC_raw32/1
  [VDDM_FCM3RCErrDTC_raw32] -> VDDM_FCM3RCErrDTC_raw32/1
  [VDDM_BMSSigErrDetDTC_raw32] -> VDDM_BMSSigErrDetDTC_raw32/1
  [VDDM_ZoneSCPNoComDTC_raw32] -> VDDM_ZoneSCPNoComDTC_raw32/1
  [VDDM_FrMCUSigErrDetDTC_raw32] -> VDDM_FrMCUSigErrDetDTC_raw32/1
  [VDDM_CCUSigErrDetDTC_raw32] -> VDDM_CCUSigErrDetDTC_raw32/1
  [VDDM_FCMACCSigErrDetDTC_raw32] -> VDDM_FCMACCSigErrDetDTC_raw32/1
  [VDDM_RrMCUSigErrDetDTC_raw32] -> VDDM_RrMCUSigErrDetDTC_raw32/1
  [VDDM_ACCMalfuncDetDTC_raw32] -> VDDM_ACCMalfuncDetDTC_raw32/1
  [VDDM_MSAMalfuncDetDTC_raw32] -> VDDM_MSAMalfuncDetDTC_raw32/1
  [VDDM_ACCAccelCmdErrDetDTC_raw32] -> VDDM_ACCAccelCmdErrDetDTC_raw32/1
  [VDDM_CCMalfuncDetDTC_raw32] -> VDDM_CCMalfuncDetDTC_raw32/1
  [VDDM_ISAMalfuncDetDTC_raw32] -> VDDM_ISAMalfuncDetDTC_raw32/1
  [VDDM_VCUACCErr_flg] -> VDDM_VCUACCErr_flg/1
  [VDDM_VCUISAErr_flg] -> VDDM_VCUISAErr_flg/1
  [VDDM_ZoneSCPNoCom_flg] -> ZoneSCP/2(VDDM_ZoneSCPNoCom_flg)
  [task_time_s] -> ZoneSCP/1(task_time_s)
  [DTC_clear_request] -> ZoneSCP/6(DTC_clear_request)
  ZoneSCP/1(VDDM_ZoneSCPNoComDFS_flg) -> Goto48/1
  ZoneSCP/2(VDDM_ZoneSCPNoComCFS_flg) -> [VDDM_ZoneSCPNoComCFS_flg]
  [No_CAN_BUS_OFF] -> ZoneSCP/3(No_CAN_BUS_OFF)
  [VINP_VehSpeed_kph] -> ZoneSCP/5(VINP_VehSpeed_kph)
  [VPMM_PowerSta_enum] -> ZoneSCP/4(VPMM_PowerSta_enum)
  Constant5/1 -> Switch2/3
  Constant4/1 -> Switch2/1
  Switch2/1 -> Goto50/1, [VDDM_EDriveSysErrVCUErrVMC_flg]
  [VDDM_ZoneSCPNoComCFS_flg] -> Switch2/2
  VDDM_ZoneSCPNoCom_flg/1 -> [VDDM_ZoneSCPNoCom_flg]
  VINP_VehSpeed_kph/1 -> [VINP_VehSpeed_kph]
  [VDDM_EDriveSysErrVCUErrVMC_flg] -> VDDM_EDriveSysErrVMC_flg/1
  FCMACC Signal Error/1(VDDM_FCMACCSigErrCFS_flg) -> [VDDM_FCMACCSigErrCFS_flg]
  [No_CAN_BUS_OFF] -> FCMACC Signal Error/4(No_CAN_BUS_OFF)
  [VPMM_PowerSta_enum] -> FCMACC Signal Error/5(VPMM_PowerSta_enum)
  [task_time_s] -> FCMACC Signal Error/1(task_time_s)
  [DTC_clear_request] -> FCMACC Signal Error/7(DTC_clear_request)
  [VDDM_FCM4NoComCFS_flg] -> FCMACC Signal Error/2(VDDM_FCM4NoComCFS_flg)
  [VDDM_FCM4CSErrCFS_flg] -> FCMACC Signal Error/3(VDDM_FCM4CSErrCFS_flg)
  [VINP_ADASACCSta_enum] -> FCMACC Signal Error/6(VINP_ADASACCSta_enum)
  [No_CAN_BUS_OFF] -> MCU_Fr Signal Error/5(No_CAN_BUS_OFF)
  [VDDM_MCUF1CSErrCFS_flg] -> MCU_Fr Signal Error/4(VDDM_MCUF1CSErrCFS_flg)
  [task_time_s] -> MCU_Fr Signal Error/1(task_time_s)
  [VPMM_PowerSta_enum] -> MCU_Fr Signal Error/6(VPMM_PowerSta_enum)
  [VDDM_MCUF1RCErrCFS_flg] -> MCU_Fr Signal Error/3(VDDM_MCUF1RCErrCFS_flg)
  [VINP_MCUWarnF_enum] -> MCU_Fr Signal Error/7(VINP_MCUWarnF_enum)
  [VDDM_MCUF1NoComCFS_flg] -> MCU_Fr Signal Error/2(VDDM_MCUF1NoComCFS_flg)
  [DTC_clear_request] -> MCU_Fr Signal Error/8(DTC_clear_request)
  MCU_Fr Signal Error/1(VDDM_FrMCUSigErrCFS_flg) -> [VDDM_FrMCUSigErrCFS_flg]
  VDDM_MCUF1NoComCFS_flg/1 -> [VDDM_MCUF1NoComCFS_flg]
  VDDM_MCUF1RCErrCFS_flg/1 -> [VDDM_MCUF1RCErrCFS_flg]
  VDDM_MCUF1CSErrCFS_flg/1 -> [VDDM_MCUF1CSErrCFS_flg]
  VINP_MCUWarnF_enum/1 -> [VINP_MCUWarnF_enum]
  [No_CAN_BUS_OFF] -> MCU_Rr Signal Error/5(No_CAN_BUS_OFF)
  [DTC_clear_request] -> MCU_Rr Signal Error/8(DTC_clear_request)
  [VDDM_MCUR1CSErrCFS_flg] -> MCU_Rr Signal Error/4(VDDM_MCUF1CSErrCFS_flg)
  [VINP_MCUWarnR_enum] -> MCU_Rr Signal Error/7(VINP_MCUWarnR_enum)
  [VPMM_PowerSta_enum] -> MCU_Rr Signal Error/6(VPMM_PowerSta_enum)
  MCU_Rr Signal Error/1(VDDM_RrMCUSigErrCFS_flg) -> [VDDM_RrMCUSigErrCFS_flg]
  [VDDM_MCUR1NoComCFS_flg] -> MCU_Rr Signal Error/2(VDDM_MCUF1NoComCFS_flg)
  [VDDM_MCUR1RCErrCFS_flg] -> MCU_Rr Signal Error/3(VDDM_MCUF1RCErrCFS_flg)
  [task_time_s] -> MCU_Rr Signal Error/1(task_time_s)
  VINP_MCUWarnR_enum/1 -> [VINP_MCUWarnR_enum]
  VDDM_MCUR1NoComCFS_flg/1 -> [VDDM_MCUR1NoComCFS_flg]
  VDDM_MCUR1RCErrCFS_flg/1 -> [VDDM_MCUR1RCErrCFS_flg]
  VDDM_MCUR1CSErrCFS_flg/1 -> [VDDM_MCUR1CSErrCFS_flg]
  [No_CAN_BUS_OFF] -> CCU Signal Error/5(No_CAN_BUS_OFF)
  [VPMM_PowerSta_enum] -> CCU Signal Error/6(VPMM_PowerSta_enum)
  [DTC_clear_request] -> CCU Signal Error/8(DTC_clear_request)
  [VDDM_C3CCU2CSCFS_flg] -> CCU Signal Error/4(VDDM_C3CCU2CSCFS_flg)
  [VDDM_C3CCU2RCCFS_flg] -> CCU Signal Error/3(VDDM_C3CCU2RCCFS_flg)
  [VINP_DCDCFaultSta_enum] -> CCU Signal Error/7(VINP_DCDCFaultSta_enum)
  [task_time_s] -> CCU Signal Error/1(task_time_s)
  [VDDM_C3CCU2LCCFS_flg] -> CCU Signal Error/2(VDDM_C3CCU2LCCFS_flg)
  CCU Signal Error/1(VDDM_CCUSigErrCFS_flg) -> [VDDM_CCUSigErrCFS_flg]
  VDDM_C3CCU2LCCFS_flg/1 -> [VDDM_C3CCU2LCCFS_flg]
  VDDM_C3CCU2RCCFS_flg/1 -> [VDDM_C3CCU2RCCFS_flg]
  VDDM_C3CCU2CSCFS_flg/1 -> [VDDM_C3CCU2CSCFS_flg]
  VINP_DCDCFaultSta_enum/1 -> [VINP_DCDCFaultSta_enum]
  [task_time_s] -> ACC Acceleration Command Error/1(task_time_s)
  [VDDM_FCM2CSErrCFS_flg] -> ACC Acceleration Command Error/4(VDDM_FCM2CSErrCFS_flg)
  [VDDM_FCM2RCErrCFS_flg] -> ACC Acceleration Command Error/3(VDDM_FCM2RCErrCFS_flg)
  [VINP_ACCRequireAccel_mps2] -> ACC Acceleration Command Error/8(VINP_ACCRequireAccel_mps2)
  [VDDM_FCM2NoComCFS_flg] -> ACC Acceleration Command Error/2(VDDM_FCM2NoComCFS_flg)
  [DTC_clear_request] -> ACC Acceleration Command Error/10(DTC_clear_request)
  [VPMM_PowerSta_enum] -> ACC Acceleration Command Error/7(VPMM_PowerSta_enum)
  [No_CAN_BUS_OFF] -> ACC Acceleration Command Error/6(No_CAN_BUS_OFF)
  ACC Acceleration Command Error/1(VDDM_ACCAccelCmdErrCFS_flg) -> [VDDM_ACCAccelCmdErrCFS_flg]
  [VVMC_ADASActive_flg] -> ACC Acceleration Command Error/5(VVMC_ADASActive_flg)
  [VINP_ADASACCSta_enum] -> ACC Acceleration Command Error/9(VINP_ADASACCSta_enum)
  [VDDM_ACCAccelCmdErrCFS_flg] -> Logical Operator2/6
  VVMC_ADASActive_flg/1 -> [VVMC_ADASActive_flg]
  VINP_ACCRequireAccel_mps2/1 -> [VINP_ACCRequireAccel_mps2]
  "ACC Malfunction "/1(VDDM_ACCMalfuncCFS_flg) -> [VDDM_ACCMalfuncCFS_flg]
  [task_time_s] -> "ACC Malfunction "/1(task_time_s)
  [No_CAN1_BUS_OFF] -> "ACC Malfunction "/29(No_CAN1_BUS_OFF)
  [No_CAN3_BUS_OFF] -> "ACC Malfunction "/30(No_CAN3_BUS_OFF)
  [No_CAN4_BUS_OFF] -> "ACC Malfunction "/31(No_CAN4_BUS_OFF)
  [VPMM_PowerSta_enum] -> "ACC Malfunction "/32(VPMM_PowerSta_enum)
  [DTC_clear_request] -> "ACC Malfunction "/34(DTC_clear_request)
  [VINP_ZoneSpdCtrlMode_enum] -> "ACC Malfunction "/33(VINP_ZoneSpdCtrlMode_enum)
  [VDDM_FCM2NoComCFS_flg] -> "ACC Malfunction "/8(VDDM_FCM2NoComCFS_flg)
  [VDDM_FCM2RCErrCFS_flg] -> "ACC Malfunction "/9(VDDM_FCM2RCErrCFS_flg)
  [VDDM_FCM2CSErrCFS_flg] -> "ACC Malfunction "/10(VDDM_FCM2CSErrCFS_flg)
  [VDDM_ACCAccelCmdErrCFS_flg] -> "ACC Malfunction "/3(VDDM_ACCAccelCmdErrCFS_flg)
  [VDDM_FCMACCSigErrCFS_flg] -> "ACC Malfunction "/2(VDDM_FCMACCSigErrCFS_flg)
  [VDDM_BMSSigErrCFS_flg] -> "ACC Malfunction "/4(VDDM_BMSSigErrCFS_flg)
  [VDDM_FrMCUSigErrCFS_flg] -> "ACC Malfunction "/5(VDDM_FrMCUSigErrCFS_flg)
  [VDDM_RrMCUSigErrCFS_flg] -> "ACC Malfunction "/6(VDDM_RrMCUSigErrCFS_flg)
  [VDDM_CCUSigErrCFS_flg] -> "ACC Malfunction "/7(VDDM_CCUSigErrCFS_flg)
  [VDDM_FCM4NoComCFS_flg] -> "ACC Malfunction "/11(VDDM_FCM4NoComCFS_flg)
  [VDDM_FCM4CSErrCFS_flg] -> "ACC Malfunction "/12(VDDM_FCM4CSErrCFS_flg)
  [VDDM_ZoneSCPNoComCFS_flg] -> "ACC Malfunction "/13(VDDM_ZoneSCPNoComCFS_flg)
  [VDDM_MCUF1CSErrCFS_flg] -> "ACC Malfunction "/19(VDDM_MCUF1CSErrCFS_flg)
  [VDDM_MCUF1RCErrCFS_flg] -> "ACC Malfunction "/18(VDDM_MCUF1RCErrCFS_flg)
  [VDDM_MCUF1NoComCFS_flg] -> "ACC Malfunction "/17(VDDM_MCUF1NoComCFS_flg)
  [VDDM_MCUR1NoComCFS_flg] -> "ACC Malfunction "/14(VDDM_MCUR1NoComCFS_flg)
  [VDDM_MCUR1RCErrCFS_flg] -> "ACC Malfunction "/15(VDDM_MCUR1RCErrCFS_flg)
  [VDDM_MCUR1CSErrCFS_flg] -> "ACC Malfunction "/16(VDDM_MCUR1CSErrCFS_flg)
  [VDDM_ESC7NoComCFS_flg] -> "ACC Malfunction "/20(VDDM_ESC7NoComCFS_flg)
  [VDDM_ESC7RCErrCFS_flg] -> "ACC Malfunction "/21(VDDM_ESC7RCErrCFS_flg)
  [VDDM_ESC7CSErrCFS_flg] -> "ACC Malfunction "/22(VDDM_ESC7CSErrCFS_flg)
  [VDDM_ESC1NoComCFS_flg] -> "ACC Malfunction "/23(VDDM_ESC1NoComCFS_flg)
  [VDDM_ESC1RCErrCFS_flg] -> "ACC Malfunction "/24(VDDM_ESC1RCErrCFS_flg)
  [VDDM_ESC1CSErrCFS_flg] -> "ACC Malfunction "/25(VDDM_ESC1CSErrCFS_flg)
  [VDDM_ESC5NoComCFS_flg] -> "ACC Malfunction "/26(VDDM_ESC5NoComCFS_flg)
  [VDDM_ESC5RCErrCFS_flg] -> "ACC Malfunction "/27(VDDM_ESC5RCErrCFS_flg)
  [VDDM_ESC5CSErrCFS_flg] -> "ACC Malfunction "/28(VDDM_ESC5CSErrCFS_flg)
  VDDM_ESC1NoComCFS_flg/1 -> [VDDM_ESC1NoComCFS_flg]
  VDDM_ESC1CSErrCFS_flg/1 -> [VDDM_ESC1CSErrCFS_flg]
  VDDM_ESC1RCErrCFS_flg/1 -> [VDDM_ESC1RCErrCFS_flg]
  VDDM_ESC7CSErrCFS_flg/1 -> [VDDM_ESC7CSErrCFS_flg]
  VDDM_ESC7NoComCFS_flg/1 -> [VDDM_ESC7NoComCFS_flg]
  VINP_ZoneSpdCtrlMode_enum/1 -> [VINP_ZoneSpdCtrlMode_enum]
  VDDM_ESC5NoComCFS_flg/1 -> [VDDM_ESC5NoComCFS_flg]
  VDDM_ESC7RCErrCFS_flg/1 -> [VDDM_ESC7RCErrCFS_flg]
  VDDM_ESC5RCErrCFS_flg/1 -> [VDDM_ESC5RCErrCFS_flg]
  VDDM_ESC5CSErrCFS_flg/1 -> [VDDM_ESC5CSErrCFS_flg]
  No_CAN4_BUS_OFF/1 -> [No_CAN4_BUS_OFF]
  No_CAN3_BUS_OFF/1 -> [No_CAN3_BUS_OFF]
  No_CAN1_BUS_OFF/1 -> [No_CAN1_BUS_OFF]
  [VDDM_ACCMalfuncCFS_flg] -> Logical Operator2/7
  [DTC_clear_request] -> "CC Malfunction "/27(DTC_clear_request)
  [No_CAN4_BUS_OFF] -> "CC Malfunction "/24(No_CAN4_BUS_OFF)
  [No_CAN1_BUS_OFF] -> "CC Malfunction "/22(No_CAN1_BUS_OFF)
  [VPMM_PowerSta_enum] -> "CC Malfunction "/25(VPMM_PowerSta_enum)
  [VINP_ZoneSpdCtrlMode_enum] -> "CC Malfunction "/26(VINP_ZoneSpdCtrlMode_enum)
  [No_CAN3_BUS_OFF] -> "CC Malfunction "/23(No_CAN3_BUS_OFF)
  [VDDM_ESC1NoComCFS_flg] -> "CC Malfunction "/16(VDDM_ESC1NoComCFS_flg)
  [VDDM_MCUF1CSErrCFS_flg] -> "CC Malfunction "/12(VDDM_MCUF1CSErrCFS_flg)
  [VDDM_ESC7CSErrCFS_flg] -> "CC Malfunction "/15(VDDM_ESC7CSErrCFS_flg)
  [VDDM_MCUF1NoComCFS_flg] -> "CC Malfunction "/10(VDDM_MCUF1NoComCFS_flg)
  [VDDM_MCUF1RCErrCFS_flg] -> "CC Malfunction "/11(VDDM_MCUF1RCErrCFS_flg)
  [VDDM_MCUR1CSErrCFS_flg] -> "CC Malfunction "/9(VDDM_MCUR1CSErrCFS_flg)
  [VDDM_MCUR1RCErrCFS_flg] -> "CC Malfunction "/8(VDDM_MCUR1RCErrCFS_flg)
  [VDDM_CCUSigErrCFS_flg] -> "CC Malfunction "/5(VDDM_CCUSigErrCFS_flg)
  [VDDM_MCUR1NoComCFS_flg] -> "CC Malfunction "/7(VDDM_MCUR1NoComCFS_flg)
  [VDDM_ZoneSCPNoComCFS_flg] -> "CC Malfunction "/6(VDDM_ZoneSCPNoComCFS_flg)
  [VDDM_FrMCUSigErrCFS_flg] -> "CC Malfunction "/3(VDDM_FrMCUSigErrCFS_flg)
  [VDDM_RrMCUSigErrCFS_flg] -> "CC Malfunction "/4(VDDM_RrMCUSigErrCFS_flg)
  [VDDM_BMSSigErrCFS_flg] -> "CC Malfunction "/2(VDDM_BMSSigErrCFS_flg)
  [task_time_s] -> "CC Malfunction "/1(task_time_s)
  "CC Malfunction "/1(VDDM_CCMalfuncCFS_flg) -> Goto86/1
  [VDDM_ESC5NoComCFS_flg] -> "CC Malfunction "/19(VDDM_ESC5NoComCFS_flg)
  [VDDM_ESC7RCErrCFS_flg] -> "CC Malfunction "/14(VDDM_ESC7RCErrCFS_flg)
  [VDDM_ESC1RCErrCFS_flg] -> "CC Malfunction "/17(VDDM_ESC1RCErrCFS_flg)
  [VDDM_ESC1CSErrCFS_flg] -> "CC Malfunction "/18(VDDM_ESC1CSErrCFS_flg)
  [VDDM_ESC7NoComCFS_flg] -> "CC Malfunction "/13(VDDM_ESC7NoComCFS_flg)
  [VDDM_ESC5RCErrCFS_flg] -> "CC Malfunction "/20(VDDM_ESC5RCErrCFS_flg)
  [VDDM_ESC5CSErrCFS_flg] -> "CC Malfunction "/21(VDDM_ESC5CSErrCFS_flg)
  [VDDM_ESC1CSErrCFS_flg] -> "MSA Malfunction "/18(VDDM_ESC1CSErrCFS_flg)
  [No_CAN1_BUS_OFF] -> "MSA Malfunction "/22(No_CAN1_BUS_OFF)
  [VDDM_ESC7NoComCFS_flg] -> "MSA Malfunction "/13(VDDM_ESC7NoComCFS_flg)
  [VDDM_RrMCUSigErrCFS_flg] -> "MSA Malfunction "/4(VDDM_RrMCUSigErrCFS_flg)
  [VPMM_PowerSta_enum] -> "MSA Malfunction "/25(VPMM_PowerSta_enum)
  [VDDM_MCUF1CSErrCFS_flg] -> "MSA Malfunction "/12(VDDM_MCUF1CSErrCFS_flg)
  [VINP_ZoneSpdCtrlMode_enum] -> "MSA Malfunction "/26(VINP_ZoneSpdCtrlMode_enum)
  [VDDM_ZoneSCPNoComCFS_flg] -> "MSA Malfunction "/6(VDDM_ZoneSCPNoComCFS_flg)
  [No_CAN4_BUS_OFF] -> "MSA Malfunction "/24(No_CAN4_BUS_OFF)
  [VDDM_MCUR1RCErrCFS_flg] -> "MSA Malfunction "/8(VDDM_MCUR1RCErrCFS_flg)
  [VDDM_ESC7CSErrCFS_flg] -> "MSA Malfunction "/15(VDDM_ESC7CSErrCFS_flg)
  [DTC_clear_request] -> "MSA Malfunction "/27(DTC_clear_request)
  [No_CAN3_BUS_OFF] -> "MSA Malfunction "/23(No_CAN3_BUS_OFF)
  [VDDM_MCUF1NoComCFS_flg] -> "MSA Malfunction "/10(VDDM_MCUF1NoComCFS_flg)
  [VDDM_ESC5CSErrCFS_flg] -> "MSA Malfunction "/21(VDDM_ESC5CSErrCFS_flg)
  [VDDM_ESC5NoComCFS_flg] -> "MSA Malfunction "/19(VDDM_ESC5NoComCFS_flg)
  [VDDM_MCUR1NoComCFS_flg] -> "MSA Malfunction "/7(VDDM_MCUR1NoComCFS_flg)
  [VDDM_BMSSigErrCFS_flg] -> "MSA Malfunction "/2(VDDM_BMSSigErrCFS_flg)
  [task_time_s] -> "MSA Malfunction "/1(task_time_s)
  [VDDM_ESC1RCErrCFS_flg] -> "MSA Malfunction "/17(VDDM_ESC1RCErrCFS_flg)
  [VDDM_MCUF1RCErrCFS_flg] -> "MSA Malfunction "/11(VDDM_MCUF1RCErrCFS_flg)
  [VDDM_MCUR1CSErrCFS_flg] -> "MSA Malfunction "/9(VDDM_MCUR1CSErrCFS_flg)
  [VDDM_ESC1NoComCFS_flg] -> "MSA Malfunction "/16(VDDM_ESC1NoComCFS_flg)
  [VDDM_ESC5RCErrCFS_flg] -> "MSA Malfunction "/20(VDDM_ESC5RCErrCFS_flg)
  [VDDM_CCUSigErrCFS_flg] -> "MSA Malfunction "/5(VDDM_CCUSigErrCFS_flg)
  "MSA Malfunction "/1(VDDM_MSAMalfuncCFS_flg) -> Goto87/1
  [VDDM_ESC7RCErrCFS_flg] -> "MSA Malfunction "/14(VDDM_ESC7RCErrCFS_flg)
  [VDDM_FrMCUSigErrCFS_flg] -> "MSA Malfunction "/3(VDDM_FrMCUSigErrCFS_flg)
  [VDDM_ESC5CSErrCFS_flg] -> "ISA Malfunction "/26(VDDM_ESC5CSErrCFS_flg)
  [VDDM_ESC5NoComCFS_flg] -> "ISA Malfunction "/24(VDDM_ESC5NoComCFS_flg)
  [VDDM_ESC1RCErrCFS_flg] -> "ISA Malfunction "/22(VDDM_ESC1RCErrCFS_flg)
  [VDDM_ESC1NoComCFS_flg] -> "ISA Malfunction "/21(VDDM_ESC1NoComCFS_flg)
  [No_CAN1_BUS_OFF] -> "ISA Malfunction "/27(No_CAN1_BUS_OFF)
  [VDDM_ESC7RCErrCFS_flg] -> "ISA Malfunction "/19(VDDM_ESC7RCErrCFS_flg)
  [VDDM_ESC1CSErrCFS_flg] -> "ISA Malfunction "/23(VDDM_ESC1CSErrCFS_flg)
  [VDDM_ESC7NoComCFS_flg] -> "ISA Malfunction "/18(VDDM_ESC7NoComCFS_flg)
  [VDDM_MCUR1CSErrCFS_flg] -> "ISA Malfunction "/14(VDDM_MCUR1CSErrCFS_flg)
  [VDDM_MCUF1RCErrCFS_flg] -> "ISA Malfunction "/16(VDDM_MCUF1RCErrCFS_flg)
  [VDDM_MCUR1RCErrCFS_flg] -> "ISA Malfunction "/13(VDDM_MCUR1RCErrCFS_flg)
  [DTC_clear_request] -> "ISA Malfunction "/32(DTC_clear_request)
  [VINP_ZoneSpdCtrlMode_enum] -> "ISA Malfunction "/31(VINP_ZoneSpdCtrlMode_enum)
  [No_CAN3_BUS_OFF] -> "ISA Malfunction "/28(No_CAN3_BUS_OFF)
  [VPMM_PowerSta_enum] -> "ISA Malfunction "/30(VPMM_PowerSta_enum)
  [No_CAN4_BUS_OFF] -> "ISA Malfunction "/29(No_CAN4_BUS_OFF)
  [VDDM_RrMCUSigErrCFS_flg] -> "ISA Malfunction "/4(VDDM_RrMCUSigErrCFS_flg)
  [VDDM_CCUSigErrCFS_flg] -> "ISA Malfunction "/5(VDDM_CCUSigErrCFS_flg)
  [VDDM_FrMCUSigErrCFS_flg] -> "ISA Malfunction "/3(VDDM_FrMCUSigErrCFS_flg)
  [VDDM_BMSSigErrCFS_flg] -> "ISA Malfunction "/2(VDDM_BMSSigErrCFS_flg)
  [VDDM_MCUF1CSErrCFS_flg] -> "ISA Malfunction "/17(VDDM_MCUF1CSErrCFS_flg)
  [task_time_s] -> "ISA Malfunction "/1(task_time_s)
  [VDDM_FCM5CSErrCFS_flg] -> "ISA Malfunction "/10(VDDM_FCM5CSErrCFS_flg)
  [VDDM_FCM5NoComCFS_flg] -> "ISA Malfunction "/9(VDDM_FCM5NoComCFS_flg)
  [VDDM_MCUF1NoComCFS_flg] -> "ISA Malfunction "/15(VDDM_MCUF1NoComCFS_flg)
  [VDDM_ESC5RCErrCFS_flg] -> "ISA Malfunction "/25(VDDM_ESC5RCErrCFS_flg)
  [VDDM_ZoneSCPNoComCFS_flg] -> "ISA Malfunction "/11(VDDM_ZoneSCPNoComCFS_flg)
  [VDDM_FCM3CSErrCFS_flg] -> "ISA Malfunction "/8(VDDM_FCM3CSErrCFS_flg)
  [VDDM_MCUR1NoComCFS_flg] -> "ISA Malfunction "/12(VDDM_MCUR1NoComCFS_flg)
  [VDDM_FCM3RCErrCFS_flg] -> "ISA Malfunction "/7(VDDM_FCM3RCErrCFS_flg)
  [VDDM_FCM3NoComCFS_flg] -> "ISA Malfunction "/6(VDDM_FCM3NoComCFS_flg)
  "ISA Malfunction "/1(VDDM_ISAMalfuncCFS_flg) -> [VDDM_ISAMalfuncCFS_flg]
  [VDDM_ESC7CSErrCFS_flg] -> "ISA Malfunction "/20(VDDM_ESC7CSErrCFS_flg)
  [VDDM_ISAMalfuncCFS_flg] -> Logical Operator1/6
  FCM2/7(VDDM_FCM2NoComDTC_raw32) -> [VDDM_FCM2NoComDTC_raw32]
  FCM2/8(VDDM_FCM2RCErrDTC_raw32) -> [VDDM_FCM2RCErrDTC_raw32]
  FCM2/9(VDDM_FCM2CSErrDTC_raw32) -> [VDDM_FCM2CSErrDTC_raw32]
  FCM3/7(VDDM_FCM3NoComDTC_raw32) -> [VDDM_FCM3NoComDTC_raw32]
  FCM3/8(VDDM_FCM3RCErrDTC_raw32) -> [VDDM_FCM3RCErrDTC_raw32]
  FCM3/9(VDDM_FCM3CSErrDTC_raw32) -> [VDDM_FCM3CSErrDTC_raw32]
  FCM4/5(VDDM_FCM4NoComDTC_raw32) -> [VDDM_FCM4NoComDTC_raw32]
  FCM4/6(VDDM_FCM4CSErrDTC_raw32) -> [VDDM_FCM4CSErrDTC_raw32]
  [VDDM_FCM4NoComDTC_raw32] -> VDDM_FCM4NoComDTC_raw32/1
  [VDDM_FCM4CSErrDTC_raw32] -> VDDM_FCM4CSErrDTC_raw32/1
  FCM5/5(VDDM_FCM5NoComDTC_raw32) -> [VDDM_FCM5NoComDTC_raw32]
  FCM5/6(VDDM_FCM5CSErrDTC_raw32) -> [VDDM_FCM5CSErrDTC_raw32]
  [VDDM_FCM5NoComDTC_raw32] -> VDDM_FCM5NoComDTC_raw32/1
  [VDDM_FCM5CSErrDTC_raw32] -> VDDM_FCM5CSErrDTC_raw32/1
  ZoneSCP/3(VDDM_ZoneSCPNoComDTC_raw32) -> [VDDM_ZoneSCPNoComDTC_raw32]
  "BMS Signal Error "/2(VDDM_BMSSigErrDetDTC_raw32) -> [VDDM_BMSSigErrDetDTC_raw32]
  FCMACC Signal Error/2(VDDM_FCMACCSigErrDetDTC_raw32) -> [VDDM_FCMACCSigErrDetDTC_raw32]
  MCU_Fr Signal Error/2(VDDM_FrMCUSigErrDetDTC_raw32) -> [VDDM_FrMCUSigErrDetDTC_raw32]
  MCU_Rr Signal Error/2(VDDM_RrMCUSigErrDetDTC_raw32) -> [VDDM_RrMCUSigErrDetDTC_raw32]
  CCU Signal Error/2(VDDM_CCUSigErrDetDTC_raw32) -> [VDDM_CCUSigErrDetDTC_raw32]
  ACC Acceleration Command Error/2(VDDM_ACCAccelCmdErrDetDTC_raw32) -> [VDDM_ACCAccelCmdErrDetDTC_raw32]
  "ACC Malfunction "/2(VDDM_ACCMalfuncDetDTC_raw32) -> [VDDM_ACCMalfuncDetDTC_raw32]
  "CC Malfunction "/2(VDDM_CCMalfuncDetDTC_raw32) -> [VDDM_CCMalfuncDetDTC_raw32]
  "MSA Malfunction "/2(VDDM_MSAMalfuncDetDTC_raw32) -> [VDDM_MSAMalfuncDetDTC_raw32]
  "ISA Malfunction "/2(VDDM_ISAMalfuncDetDTC_raw32) -> [VDDM_ISAMalfuncDetDTC_raw32]

== system ddm/DDM/DDM/APM/Subsystem ==
  USSSta_flg : Inport
  VPMM_SysPwrSta_enum : Inport  Port=2
  VAPM_SNSRLayout_enum : Inport  Port=3
  Constant1 : Constant  Value=ENUM_PWRSTASW_READY
  Constant17 : Constant  Value=ENUM_PWRSTASW_READY
  Constant2 : Constant  Value=ENUM_PWRSTASW_ON
  Constant25 : Constant  Value=FALSE
  Constant3 : Constant  Value=ENUM_PWRSTASW_ON
  Constant4 : Constant  Value=ENUM_APS
  Constant5 : Constant  Value=ENUM_PAS_R2F2
  Equal{1..6} (6 alike) : RelationalOperator  Operator===  OutDataTypeStr=boolean  RndMeth=Simplest
  Logical Operator1 : Logic  Operator=NOT  AllPortsSameDT=off  OutDataTypeStr=boolean
  Logical Operator13 : Logic  Operator=OR  AllPortsSameDT=off  OutDataTypeStr=boolean
  Logical Operator2 : Logic  AllPortsSameDT=off  OutDataTypeStr=boolean
  Logical Operator3 : Logic  Operator=OR  AllPortsSameDT=off  OutDataTypeStr=boolean
  Logical Operator4 : Logic  AllPortsSameDT=off  OutDataTypeStr=boolean
  Logical Operator5 : Logic  Operator=OR  AllPortsSameDT=off  OutDataTypeStr=boolean
  Switch2 : Switch  Criteria=u2 ~= 0
  Pass_flg : Outport
  CFS_flg : Outport  Port=2
  wires:
  VPMM_SysPwrSta_enum/1 -> [VPMM_SysPwrSta_enum]
  Logical Operator4/1 -> CFS_flg/1
  Switch2/1 -> Logical Operator4/1, Logical Operator1/1
  [VPMM_SysPwrSta_enum] -> Equal1/1
  Equal3/1 -> Logical Operator3/1
  Constant1/1 -> Equal1/2
  Constant2/1 -> Equal3/2
  Equal1/1 -> Logical Operator3/2
  [VPMM_SysPwrSta_enum] -> Equal3/1
  Logical Operator3/1 -> Logical Operator4/2
  Logical Operator2/1 -> Pass_flg/1
  Logical Operator1/1 -> Logical Operator2/2
  Logical Operator13/1 -> Logical Operator2/1
  [VPMM_SysPwrSta_enum] -> Equal6/1
  Equal2/1 -> Logical Operator13/2
  Constant3/1 -> Equal6/2
  Constant17/1 -> Equal2/2
  Equal6/1 -> Logical Operator13/1
  [VPMM_SysPwrSta_enum] -> Equal2/1
  USSSta_flg/1 -> Switch2/1
  Equal4/1 -> Logical Operator5/1
  Constant25/1 -> Switch2/3
  Constant4/1 -> Equal4/1
  VAPM_SNSRLayout_enum/1 -> Equal4/2, Equal5/1
  Logical Operator5/1 -> Switch2/2
  Equal5/1 -> Logical Operator5/2
  Constant5/1 -> Equal5/2

== system ddm/DDM/DDM/APM/Subsystem1 ==
  USSSta_flg : Inport
  VPMM_SysPwrSta_enum : Inport  Port=2
  VAPM_SNSRLayout_enum : Inport  Port=3
  Constant1 : Constant  Value=ENUM_PWRSTASW_READY
  Constant17 : Constant  Value=ENUM_PWRSTASW_READY
  Constant2 : Constant  Value=ENUM_PWRSTASW_ON
  Constant25 : Constant  Value=FALSE
  Constant3 : Constant  Value=ENUM_PWRSTASW_ON
  Constant5 : Constant  Value=ENUM_APS
  Equal{1..3,5..6} (5 alike) : RelationalOperator  Operator===  OutDataTypeStr=boolean  RndMeth=Simplest
  Logical Operator1 : Logic  Operator=NOT  AllPortsSameDT=off  OutDataTypeStr=boolean
  Logical Operator13 : Logic  Operator=OR  AllPortsSameDT=off  OutDataTypeStr=boolean
  Logical Operator2 : Logic  AllPortsSameDT=off  OutDataTypeStr=boolean
  Logical Operator3 : Logic  Operator=OR  AllPortsSameDT=off  OutDataTypeStr=boolean
  Logical Operator4 : Logic  AllPortsSameDT=off  OutDataTypeStr=boolean
  Switch2 : Switch  Criteria=u2 ~= 0
  Pass_flg : Outport
  CFS_flg : Outport  Port=2
  wires:
  [VPMM_SysPwrSta_enum] -> Equal2/1
  Equal6/1 -> Logical Operator13/1
  Constant17/1 -> Equal2/2
  Constant3/1 -> Equal6/2
  Equal2/1 -> Logical Operator13/2
  [VPMM_SysPwrSta_enum] -> Equal6/1
  Logical Operator13/1 -> Logical Operator2/1
  Logical Operator1/1 -> Logical Operator2/2
  Logical Operator2/1 -> Pass_flg/1
  Logical Operator3/1 -> Logical Operator4/2
  [VPMM_SysPwrSta_enum] -> Equal3/1
  Equal1/1 -> Logical Operator3/2
  Constant2/1 -> Equal3/2
  Constant1/1 -> Equal1/2
  Equal3/1 -> Logical Operator3/1
  [VPMM_SysPwrSta_enum] -> Equal1/1
  Switch2/1 -> Logical Operator4/1, Logical Operator1/1
  Logical Operator4/1 -> CFS_flg/1
  VPMM_SysPwrSta_enum/1 -> [VPMM_SysPwrSta_enum]
  Constant5/1 -> Equal5/2
  VAPM_SNSRLayout_enum/1 -> Equal5/1
  Equal5/1 -> Switch2/2
  Constant25/1 -> Switch2/3
  USSSta_flg/1 -> Switch2/1
